simulink model "PID_Position_IntegralSMC_Attitude"  (R2018a)
settings: Solver=FixedStepAuto  StartTime=0.0  StopTime=60  FixedStep=1e-3  RelTol=1e-3
settings Model: Creator=hellb  LastModifiedBy=hellb

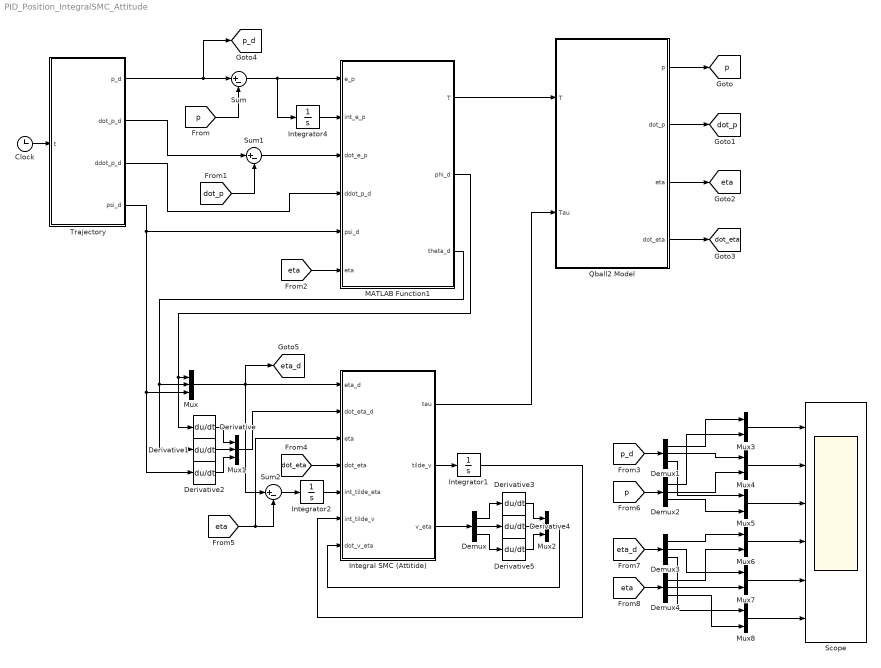
== system PID_Position_IntegralSMC_Attitude ==
  Clock : Clock
  Demux{,1..4} (5 alike) : Demux  Outputs=3
  Derivative{,1..5} (6 alike) : Derivative
  Integral SMC (Attitide) : MATLAB Function  TreatAsAtomicUnit=on
  Integrator1 : Integrator  InitialCondition=[0;0;0]
  Integrator2 : Integrator  InitialCondition=[0;0;0]
  Integrator4 : Integrator  InitialCondition=[0;0;0]
  MATLAB Function1 : MATLAB Function  TreatAsAtomicUnit=on
  Mux : Mux  Inputs=3
  Mux1 : Mux  Inputs=3
  Mux2 : Mux  Inputs=3
  Mux{3..8} (6 alike) : Mux  Inputs=2
  Qball2 Model : Subsystem
  Scope : Scope  NumInputPorts=6
  Sum : Sum  Inputs=|+-
  Sum1 : Sum  Inputs=|+-
  Sum2 : Sum  Inputs=|+-
  Trajectory : MATLAB Function  TreatAsAtomicUnit=on
  tag scope: dot_eta=global, dot_p=global, eta=global, eta_d=global, p=global, p_d=global
  wires:
  Demux1/3 -> Mux5/1
  Derivative5/1 -> Mux2/3
  Demux4/3 -> Mux8/2
  Integrator1/1 -> Integral SMC (Attitide)/6(int_tilde_v)
  Mux7/1 -> Scope/5
  Trajectory/4(psi_d) -> MATLAB Function1/5(psi_d), Derivative2/1, Mux/3
  Derivative/1 -> Mux1/1
  Demux3/3 -> Mux8/1
  Demux1/1 -> Mux3/1
  Qball2 Model/4(dot_eta) -> [dot_eta]
  Demux3/2 -> Mux7/1
  Trajectory/2(dot_p_d) -> Sum1/1
  Demux2/3 -> Mux5/2
  [p] -> Demux2/1
  Demux2/2 -> Mux4/2
  [eta] -> Integral SMC (Attitide)/3(eta), Sum2/2
  [eta] -> Demux4/1
  Demux2/1 -> Mux3/2
  Demux1/2 -> Mux4/1
  Mux2/1 -> Integral SMC (Attitide)/7(dot_v_eta)
  [dot_eta] -> Integral SMC (Attitide)/4(dot_eta)
  Demux/3 -> Derivative5/1
  Derivative4/1 -> Mux2/2
  Sum2/1 -> Integrator2/1
  Integral SMC (Attitide)/3(v_eta) -> Demux/1
  Demux/2 -> Derivative4/1
  Derivative2/1 -> Mux1/3
  Derivative1/1 -> Mux1/2
  Integral SMC (Attitide)/1(tau) -> Qball2 Model/2(Tau)
  Demux3/1 -> Mux6/1
  Demux/1 -> Derivative3/1
  Mux6/1 -> Scope/4
  [eta_d] -> Demux3/1
  [p] -> Sum/2
  Mux5/1 -> Scope/3
  Mux1/1 -> Integral SMC (Attitide)/2(dot_eta_d)
  Mux4/1 -> Scope/2
  [dot_p] -> Sum1/2
  Mux3/1 -> Scope/1
  Qball2 Model/2(dot_p) -> [dot_p]
  Integrator2/1 -> Integral SMC (Attitide)/5(int_tilde_eta)
  Clock/1 -> Trajectory/1(t)
  Qball2 Model/3(eta) -> [eta]
  Trajectory/1(p_d) -> [p_d], Sum/1
  Mux8/1 -> Scope/6
  [p_d] -> Demux1/1
  Demux4/1 -> Mux6/2
  Integral SMC (Attitide)/2(tilde_v) -> Integrator1/1
  Qball2 Model/1(p) -> [p]
  Demux4/2 -> Mux7/2
  Derivative3/1 -> Mux2/1
  Mux/1 -> [eta_d], Sum2/1, Integral SMC (Attitide)/1(eta_d)
  Integrator4/1 -> MATLAB Function1/2(int_e_p)
  MATLAB Function1/1(T) -> Qball2 Model/1(T)
  MATLAB Function1/3(theta_d) -> Derivative1/1, Mux/2
  MATLAB Function1/2(phi_d) -> Derivative/1, Mux/1
  [eta] -> MATLAB Function1/6(eta)
  Sum/1 -> Integrator4/1, MATLAB Function1/1(e_p)
  Sum1/1 -> MATLAB Function1/3(dot_e_p)
  Trajectory/3(ddot_p_d) -> MATLAB Function1/4(ddot_p_d)

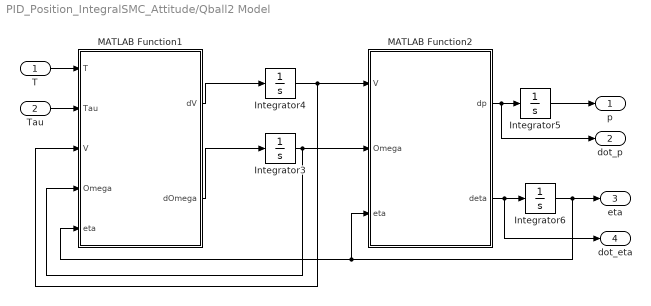
== system PID_Position_IntegralSMC_Attitude/Qball2 Model ==
  T : Inport
  Tau : Inport  Port=2
  Integrator3 : Integrator  InitialCondition=[0;0;0]
  Integrator4 : Integrator  InitialCondition=[0;0;0]
  Integrator5 : Integrator  InitialCondition=[0;0;0.3]  LimitOutput=on  UpperSaturationLimit=[inf;inf;inf]  LowerSaturationLimit=[-inf;-inf;0.3]
  Integrator6 : Integrator  InitialCondition=[0;0;0]
  MATLAB Function1 : MATLAB Function  TreatAsAtomicUnit=on
  MATLAB Function2 : MATLAB Function  TreatAsAtomicUnit=on
  p : Outport
  dot_p : Outport  Port=2
  eta : Outport  Port=3
  dot_eta : Outport  Port=4
  wires:
  MATLAB Function2/2(deta) -> Integrator6/1, dot_eta/1
  MATLAB Function2/1(dp) -> dot_p/1, Integrator5/1
  MATLAB Function1/1(dV) -> Integrator4/1
  MATLAB Function1/2(dOmega) -> Integrator3/1
  Tau/1 -> MATLAB Function1/2(Tau)
  T/1 -> MATLAB Function1/1(T)
  Integrator6/1 -> eta/1, MATLAB Function2/3(eta), MATLAB Function1/5(eta)
  Integrator5/1 -> p/1
  Integrator3/1 -> MATLAB Function1/4(Omega), MATLAB Function2/2(Omega)
  Integrator4/1 -> MATLAB Function1/3(V), MATLAB Function2/1(V)

== matlab function PID_Position_IntegralSMC_Attitude/Trajectory ==
  data: t input; p_d output; dot_p_d output; ddot_p_d output; psi_d output
function [p_d,dot_p_d,ddot_p_d,psi_d] = fcn(t)

x_amp = 0.5;
y_amp = 1;
% z_amp = 0;

x_frec = 2*pi/4;
y_frec = 2*pi/8;
% z_frec = 0;

z_b = 1;

p_d = [x_amp*sin(x_frec*t);
       y_amp*cos(y_frec*t);
       z_b];
   
dot_p_d = [x_frec*x_amp*cos(x_frec*t);
           y_frec*y_amp*-sin(y_frec*t);
           0];
       
ddot_p_d = [x_frec^2*x_amp*-sin(x_frec*t);
            y_frec^2*y_amp*-cos(y_frec*t);
            0];
        
psi_d = 0;

== matlab function PID_Position_IntegralSMC_Attitude/MATLAB Function1 ==
  data: e_p input; int_e_p input; T output; phi_d output; dot_e_p input; ddot_p_d input; psi_d input; eta input; theta_d output
function [T, phi_d, theta_d] = fcn(e_p, int_e_p, dot_e_p, ddot_p_d, psi_d, eta)

m = 1.79;
g = 9.81;

phi   = eta(1);
theta = eta(2);

e_x = e_p(1);
e_y = e_p(2);
e_z = e_p(3);

dot_e_x = dot_e_p(1);
dot_e_y = dot_e_p(2);
dot_e_z = dot_e_p(3);

int_e_x = int_e_p(1);
int_e_y = int_e_p(2);
int_e_z = int_e_p(3);

% kpx = 7; kdx = 2.5; kix = 0.1;
% kpy = kpx; kdy = kdx; kiy = kix;
% kpz = 10; kdz = 4.5; kiz = 0.01;

kpx = 3.5; kdx = 1.25; kix = 0.05;
kpy = kpx; kdy = kdx; kiy = kix;
kpz = 5; kdz = 2.25; kiz = 0.005;

nu = m*ddot_p_d(3) + m*g + kpz*e_z + kdz*dot_e_z + kiz*int_e_z;

fI1 = (m*ddot_p_d(1) + kpx*e_x + kdx*dot_e_x + kix*int_e_x);
fI2 = (m*ddot_p_d(2) + kpy*e_y + kdy*dot_e_y + kiy*int_e_y);

T      = nu/(cos(theta)*cos(phi));
theta_d = atan((fI1*cos(psi_d) + fI2*sin(psi_d))/nu);
phi_d   = atan((cos(theta_d)*(fI1*sin(psi_d) - fI2*cos(psi_d)))/nu);

== matlab function PID_Position_IntegralSMC_Attitude/Integral SMC (Attitide) ==
  data: eta_d input; dot_eta_d input; tau output; eta input; dot_eta input; int_tilde_eta input; int_tilde_v input; dot_v_eta input; tilde_v output; v_eta output
function [tau, tilde_v, v_eta]  = fcn(eta_d, dot_eta_d, eta, dot_eta, int_tilde_eta, int_tilde_v, dot_v_eta)

Ixx = 0.03;
Iyy = Ixx;
Izz = 0.04;

kw    = 100;
kn    = 20;
rho_w = 0.001;
rho_n = 0.001;

phi   = eta(1);
theta = eta(2);

dot_phi   = dot_eta(1);
dot_theta = dot_eta(2);
dot_psi   = dot_eta(3);

M_eta = [Ixx 0 -Ixx*sin(theta);
         0 Iyy*cos(phi)^2+Izz*sin(phi)^2 (Iyy-Izz)*cos(phi)*sin(phi)*cos(theta);
         -Ixx*sin(theta) (Iyy-Izz)*cos(phi)*sin(phi)*cos(theta) Ixx*sin(theta)^2+Iyy*sin(phi)^2*cos(theta)^2+Izz*cos(phi)^2*cos(theta)^2];

C12 = (Iyy-Izz)*(dot_theta*cos(phi)*sin(phi)+dot_psi*sin(phi)^2*cos(theta))...
    + (Izz-Iyy)*dot_psi*cos(phi)^2*cos(theta)...
    - Ixx*dot_psi*cos(theta);

C13 = (Izz-Iyy)*dot_psi*cos(phi)*sin(phi)*cos(theta)^2;

C21 = (Izz-Iyy)*(dot_theta*cos(phi)*sin(phi)+dot_psi*sin(phi)^2*cos(theta))...
    + (Iyy-Izz)*dot_psi*cos(phi)^2*cos(theta)...
    + Ixx*dot_psi*cos(theta);

C22 = (Izz-Iyy)*dot_phi*cos(phi)*sin(phi);

C23 = -Ixx*dot_psi*sin(theta)*cos(theta)...
    + Iyy*dot_psi*sin(phi)^2*cos(theta)*sin(theta)...
    + Izz*dot_psi*cos(phi)^2*sin(theta)*cos(theta);

C31 = (Iyy-Izz)*dot_psi*cos(theta)^2*sin(phi)*cos(phi)...
    - Ixx*dot_theta*cos(theta);

C32 = (Izz-Iyy)*(dot_theta*cos(phi)*sin(phi)*sin(theta))...
    + (Iyy-Izz)*dot_phi*cos(phi)^2*cos(theta)...
    + Ixx*dot_psi*sin(theta)*cos(theta)...
    - Iyy*dot_psi*sin(phi)^2*sin(theta)*cos(theta)...
    - Izz*dot_theta*cos(phi)^2*sin(theta)*cos(theta);

C33 = (Iyy-Izz)*dot_phi*cos(phi)*sin(phi)*cos(theta)^2 ...
    - Iyy*dot_theta*sin(phi)^2*cos(theta)*sin(theta)...
    - Izz*dot_theta*cos(phi)^2*cos(theta)*sin(theta)...
    + Ixx*dot_theta*cos(theta)*sin(theta);

C_eta = [0   C12 C13;
         C21 C22 C23;
         C31 C32 C33];
     
tilde_eta = eta_d - eta;

s_w = tilde_eta + kw*int_tilde_eta;

v_eta = dot_eta_d + kw*tilde_eta + rho_w*sign(s_w);

tilde_v = v_eta - dot_eta;
     
s_n = tilde_v + kn*int_tilde_v;
     
tau = M_eta*dot_v_eta + C_eta*dot_eta + rho_n*sign(s_n) + kn*M_eta*tilde_v;

== matlab function PID_Position_IntegralSMC_Attitude/Qball2 Model/MATLAB Function1 ==
  data: T input; Tau input; V input; dV output; Omega input; eta input; dOmega output
function [dV,dOmega] = fcn(T,Tau,V,Omega,eta)

%  TTA = [1.7613 %Parametros identificados 1
%     0.0128
%     0.0151
%     0.0024];

%  TTA = [1.7874 %Parametros identificados 2
%     0.0156
%     0.0186
%     0.0010];

%  TTA = [1.7917 %Parametros identificados 3
%     0.0140
%     0.0148
%     0.0013];

 TTA = [1.79 %Parametros fabricante
    0.03
    0.03
    0.04];

TAUphi = Tau(1);
TAUtta = Tau(2);
TAUpsi = Tau(3);

u = V(1);
v = V(2);
w = V(3);

p = Omega(1);
q = Omega(2);
r = Omega(3);

phi = eta(1);
tta = eta(2);

gbx = -9.8*sin(tta);
gby = 9.8*cos(tta)*sin(phi);
gbz = 9.8*cos(tta)*cos(phi);

  m = TTA(1,1);
Ixx = TTA(2,1);
Iyy = TTA(3,1);
Izz = TTA(4,1);

du = r*v - q*w - gbx;
dv = p*w - r*u - gby;
dw = q*u - p*v - gbz + T/m;
dp = ((Iyy-Izz)*q*r + TAUphi)/Ixx;
dq = ((Izz-Ixx)*p*r + TAUtta)/Iyy;
dr = ((Ixx-Iyy)*p*q + TAUpsi)/Izz;

    dV = [du;dv;dw];
dOmega = [dp;dq;dr];

== matlab function PID_Position_IntegralSMC_Attitude/Qball2 Model/MATLAB Function2 ==
  data: V input; dp output; Omega input; eta input; deta output
function [dp,deta] = fcn(V,Omega,eta)

phi = eta(1);
tta = eta(2);
psi = eta(3);

R = [cos(psi)*cos(tta)  -sin(psi)*cos(phi)+cos(psi)*sin(tta)*sin(phi)   sin(psi)*sin(phi)+cos(psi)*cos(phi)*sin(tta)
     sin(psi)*cos(tta)   cos(psi)*cos(phi)+sin(phi)*sin(tta)*sin(psi)   sin(tta)*sin(psi)*cos(phi)-cos(psi)*sin(phi)
     -sin(tta)           cos(tta)*sin(phi)                              cos(tta)*cos(phi)];
 
W = [1  sin(phi)*tan(tta)   cos(phi)*tan(tta)
     0  cos(phi)           -sin(phi)
     0  sin(phi)/cos(tta)   cos(phi)/cos(tta)];

dp = R*V;
deta = W*Omega;
